simulink model "trackAnimationSim"  (R2026a)
settings: Solver=VariableStepAuto
settings Model: Creator=jason  LastModifiedBy=jason

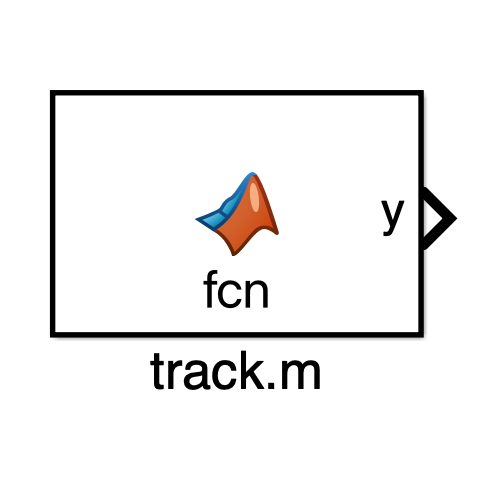
[thumbnail: Simulink's stored preview of the top-level diagram]
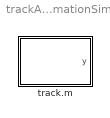
== system trackAnimationSim ==
  track.m : MATLAB Function  TreatAsAtomicUnit=on

== matlab function trackAnimationSim/track.m ==
  data: y output
function y = fcn()
    coder.extrinsic('evalin');
    persistent done
    if isempty(done)
        done = false;
    end

    y = 0;

    % runs only once
    if ~done 
        evalin('base', 'track');
        done = true;
    end
end
